simulink library "WBCLibrary"  (Simulink 7.9)
settings: Solver=ode45  StartTime=0.0  StopTime=10.0  RelTol=1e-3
undefined symbols (not defined in the file or in its folder): localName, robotName
libraries: WBCLibrary x5, dspmtrx3 x3, simulink x1, dspsigops x1
settings Model: ForwardingTableString=||__slOldName__||WBCLibrary/wholeBodyModel/Jacobians/COM Jacobian||__slNewName__||WBCLibrary/wholeBodyModel/Jacobians/Center of Mass Jacobian||__slOldName__||WBCLibrary/wholeBodyModel/Jacobians/Right Foot Jacobian1||__slNewName__||WBCLibrary/wholeBodyModel/Jacobians/Right Foot Jacobian||__slOldName__||WBCLibrary/wholeBodyActuators/setVelDes1||__slNewName__||WBCLibrary/wholeBodyActuators/Set Velocities||__slOldName__||WBCLibrary/wholeBodyActuators/setVelDes||__slNewName__||WBCLibrary/wholeBodyActuators/Set Velocities  Creator=jorhabib  LastModifiedBy=jorhabib

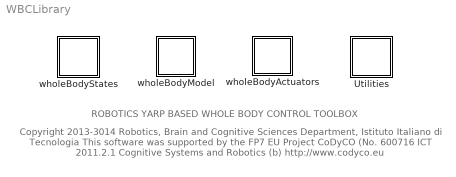
== system WBCLibrary ==
  note: ROBOTICS YARP BASED WHOLE BODY CONTROL TOOLBOX
  note: Copyright  2013-3014 Robotics, Brain and Cognitive Sciences Department, Istituto Italiano di Tecnologia
      | This software was supported by the FP7 EU Project CoDyCO (No. 600716 ICT 2011.2.1 Cognitive Systems and Robotics (b)
      | http://www.codyco.eu
  Utilities : Subsystem
      mask Display: image(imread('utilities.bmp'))
  wholeBodyActuators : Subsystem
      mask Display: image(imread('wholeBodyActuators.bmp'),'center')
  wholeBodyModel : Subsystem
      mask Display: image(imread('wholeBodyModel.bmp'),'center')
  wholeBodyStates : Subsystem
      mask Display: image(imread('wholeBodyStates.bmp'),'center');

== system WBCLibrary/Utilities ==
  DampPinv : Subsystem  mask{tol=1e-4}
      mask prompts: tol "Tolerance"
  S-Function : S-Function  FunctionName=sfun_time  Parameters=rate  EnableBusSupport=off  mask(Soft Real Time){rate=0.010}
      mask prompts: rate "Simulation rate"
      mask Display: disp('SoftRealTime')
  TruncPinv : Subsystem  mask{tol=1e-4}
      mask prompts: tol "Tolerance"
  WBI to yarp : Subsystem
  baseVelocity : Subsystem
      mask Type: baseVelocity
      mask Description: This block computes the velocity of the floating base of a bipedal robot
  errors : Subsystem
  holder : Subsystem
  minJerkTrajGen : Subsystem
      mask Type: minJerkTrajGen
      mask Description:
      | This block wraps the minJerkTrajGen class from iCub::ctrl::minJerkTrajGen.
      | 
      | The min jerk trajectory is approximated using a 3rd order LTI dynamical system (for more details see Pattacini2010). Position, velocity and acceleration trajectories are computed. The main advantage with respect to the standard polynomial form is that if the reference value yd changes there is no need to recompute the filter coefficients.
  yarp read : S-Function  FunctionName=yRead  Parameters=from,to,num  EnableBusSupport=off  mask{from=['/' robotName '/torso/state:o'], to='...', num=3}
  yarp to WBI : Subsystem
  yarp write : Subsystem  mask{port_name='...'}
      mask prompts: port_name "Specify port name starting with "/" e.g. '/port/input:i'"

== system WBCLibrary/wholeBodyActuators ==
  note: DO NOT USE YET.
      | UNDER DEVELOPMENT
  ControlMode : Subsystem  mask{ctrlMode=Velocity}
      mask prompts: ctrlMode "Control Mode"
      mask init:
      | switch ctrlMode
      |     case 'Velocity'
      | %         display('Velocity Mode selected')
      |         current = gcb;
      |         block = find_system(current,...
      |             'LookUnderMasks','on',...
      |             'FollowLinks','on','Name','set Velocities');
      |         if ~isempty(block)
      | %             display('setVelDes will be deleted')
      |             delete_block(block)
      | %             display('setVelDes has been deleted')
      |             add_block('WBCLibrary/wholeBodyActuators/set Velocities', [current,'/setVelDes1'])            
      | %             display('New setVelDes has been created')
      |             add_line(current,'In1/1',[current '/set Velocities/1'])
      |         else
      | %             display('A new setVelDes will be created')
      |             add_block('WBCLibrary/wholeBodyActuators/set Velocities', [current,'/setVelDes1'])            
      |         end
      | end
      mask StyleString: popup(Position|Velocity|Torque)
  Set Angles : Subsystem  mask{val=5, robotName=robotName, localName=localName}
      mask prompts: val "Block type"; robotName "Robot name"; localName "Local name"
  Set Torques : Subsystem  mask{val=6, robotName=robotName, localName=localName}
      mask prompts: val "Block type"; robotName "Robot name"; localName "Local name"
  Set Velocities : Subsystem  mask{val=4, robotName=robotName, localName=localName}
      mask prompts: val "Block type"; robotName "Robot name"; localName "Local name"

== system WBCLibrary/wholeBodyModel ==
  Dynamics : Subsystem
      mask Display: image(imread('dynamics.jpg'))
  Forward Kinematics : Subsystem
      mask Display: image(imread('rightLeg.jpg'))
  Jacobians : Subsystem
      mask Display: image(imread('jacobian.png'))
  Joint Limits : Subsystem  mask{robotName=robotName, localName=localName}
      mask prompts: robotName "Robot name"; localName "Local name"

== system WBCLibrary/wholeBodyStates ==
  DUMMY Joint Torques : Subsystem  mask{robotName=robotName, localName=localName}
      mask prompts: robotName "Robot name"; localName "Local name"
      mask Display: disp('dummy tau')
  Joint Accelerations : Subsystem  mask(Get Joint Accelerations){robotName=robotName, localName=localName}
      mask prompts: robotName "Robot name"; localName "Local name"
      mask Display: disp('ddq')
  Joint Angles : Subsystem  mask{robotName=robotName, localName=localName}
      mask Display: disp('q')
  Joint Torques : Subsystem  mask(Get Joint Torques){robotName=robotName, localName=localName}
      mask prompts: robotName "Robot name"; localName "Local name"
      mask Display: disp('tau')
  Joint Velocities : Subsystem  mask{robotName=robotName, localName=localName}
      mask Display: disp('dq')

== system WBCLibrary/Utilities/DampPinv ==
  mat : Inport
  sigma : Inport  Port=2
  Damped Pseudo Inverse : MATLAB Function  TreatAsAtomicUnit=on
  DPinv : Outport
  wires:
  sigma/1 -> Damped Pseudo Inverse/2(sigma)
  Damped Pseudo Inverse/1(DPinv) -> DPinv/1
  mat/1 -> Damped Pseudo Inverse/1(mat)

== system WBCLibrary/Utilities/TruncPinv ==
  S : Inport
  tol : Inport  Port=2
  Truncated PseudoInverse : MATLAB Function  TreatAsAtomicUnit=on
  Tpinv : Outport
  wires:
  S/1 -> Truncated PseudoInverse/1(mat)
  Truncated PseudoInverse/1(TPinv) -> Tpinv/1
  tol/1 -> Truncated PseudoInverse/2(tol)

== system WBCLibrary/Utilities/WBI to yarp ==
  WBI ordered : Inport
  Selector : Selector  InputPortWidth=25  IndexOptions=Index vector (dialog)  Indices=[1 2 3]  OutputSizes=1
  Selector1 : Selector  InputPortWidth=25  IndexOptions=Index vector (dialog)  Indices=[4 5 6 7 8]  OutputSizes=1
  Selector2 : Selector  InputPortWidth=25  IndexOptions=Index vector (dialog)  Indices=[9 10 11 12 13]  OutputSizes=1
  Selector3 : Selector  InputPortWidth=25  IndexOptions=Index vector (dialog)  Indices=[14 15 16 17 18 19]  OutputSizes=1
  Selector4 : Selector  InputPortWidth=25  IndexOptions=Index vector (dialog)  Indices=[20 21 22 23 24 25]  OutputSizes=1
  Selector5 : Selector  InputPortWidth=3  IndexOptions=Index vector (dialog)  Indices=[3 2 1]  OutputSizes=1
  torso : Outport
  leftArm : Outport  Port=2
  rightArm : Outport  Port=3
  leftLeg : Outport  Port=4
  rightLeg : Outport  Port=5
  wires:
  Selector1/1 -> leftArm/1
  Selector2/1 -> rightArm/1
  Selector3/1 -> leftLeg/1
  Selector4/1 -> rightLeg/1
  WBI ordered/1 -> Selector/1, Selector1/1, Selector2/1, Selector4/1, Selector3/1
  Selector/1 -> Selector5/1
  Selector5/1 -> torso/1

== system WBCLibrary/Utilities/baseVelocity ==
  JacobRF : Inport
  JacobLF : Inport  Port=2
  dq : Inport  Port=3
  MATLAB Function : MATLAB Function  TreatAsAtomicUnit=on
  baseVel : Outport
  wires:
  dq/1 -> MATLAB Function/3(qD)
  MATLAB Function/1(y) -> baseVel/1
  JacobRF/1 -> MATLAB Function/1(JacobRF)
  JacobLF/1 -> MATLAB Function/2(JacobLF)

== system WBCLibrary/Utilities/errors ==
  x : Inport
  y : Inport  Port=2
  Add : Sum  Inputs=+-
  Divide : Product  Inputs=*/
  x-y : Outport
  (x-y)./y : Outport  Port=2
  wires:
  Add/1 -> Divide/1, x-y/1
  x/1 -> Add/1
  y/1 -> Add/2, Divide/2
  Divide/1 -> (x-y)./y/1

== system WBCLibrary/Utilities/holder ==
  s : Inport
  Clock : Clock
  Compare To Constant : simulink/Logic and Bit Operations/Compare To Constant  relop===  const=0  OutDataTypeStr=boolean
  Memory : Memory
  Sample and Hold : dspsigops/Sample and Hold  trig=Falling edge  initCond=0  latchinput=off
  Switch : Switch  Criteria=u2 > Threshold
  s(0) : Outport
  wires:
  s/1 -> Switch/1, Memory/1
  Clock/1 -> Compare To Constant/1
  Compare To Constant/1 -> Sample and Hold/Trigger, Switch/2
  Sample and Hold/1 -> Switch/3
  Switch/1 -> s(0)/1
  Memory/1 -> Sample and Hold/1

== system WBCLibrary/Utilities/minJerkTrajGen ==
  desiredPos : Inport
  initPos : Inport  Port=2
  S-Function : S-Function  FunctionName=minJerkGenerator  Parameters=dim, rate, tt  EnableBusSupport=off  mask{dim=25, rate=10, tt=4}
      mask prompts: dim "Trajectory dimension (int)"; rate "Simulation rate (int) [ms]"; tt "Trajectory time [s]"
  pos : Outport
  vel : Outport  Port=2
  acc : Outport  Port=3
  wires:
  desiredPos/1 -> S-Function/2
  initPos/1 -> S-Function/1
  S-Function/3 -> acc/1
  S-Function/1 -> pos/1
  S-Function/2 -> vel/1

== system WBCLibrary/Utilities/yarp to WBI ==
  torso : Inport
  leftArm : Inport  Port=2
  rightArm : Inport  Port=3
  leftLeg : Inport  Port=4
  rightLeg : Inport  Port=5
  Mux3 : Mux  Inputs=5
  Selector : Selector  InputPortWidth=3  IndexOptions=Index vector (dialog)  Indices=[3 2 1]  OutputSizes=1
  WBI ordered : Outport
  wires:
  Selector/1 -> Mux3/1
  torso/1 -> Selector/1
  leftArm/1 -> Mux3/2
  rightArm/1 -> Mux3/3
  Mux3/1 -> WBI ordered/1
  leftLeg/1 -> Mux3/4
  rightLeg/1 -> Mux3/5

== system WBCLibrary/Utilities/yarp write ==
  In1 : Inport
  S-Function : S-Function  FunctionName=yWrite  Parameters=port_name  EnableBusSupport=off
  wires:
  In1/1 -> S-Function/1

== system WBCLibrary/wholeBodyActuators/ControlMode ==
  In1 : Inport

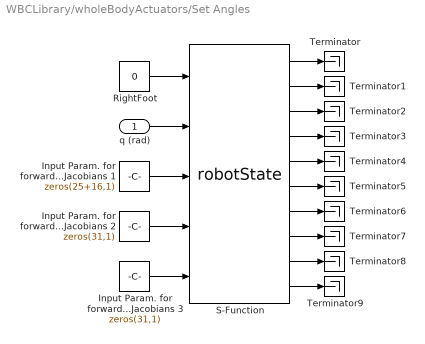
== system WBCLibrary/wholeBodyActuators/Set Angles ==
  q (rad) : Inport
  Input Param. for forwardKinematics and  computeJacobians 1 : Constant  Value=zeros(25+16,1)  OutDataTypeStr=double  SampleTime=-1
  Input Param. for forwardKinematics and  computeJacobians 2 : Constant  Value=zeros(31,1)  OutDataTypeStr=double  SampleTime=-1
  Input Param. for forwardKinematics and  computeJacobians 3 : Constant  Value=zeros(31,1)  OutDataTypeStr=double  SampleTime=-1
  RightFoot : Constant  Value=0  OutDataTypeStr=int8  SampleTime=-1
  S-Function : S-Function  FunctionName=robotState  Parameters=val,robotName,localName  EnableBusSupport=off
  Terminator{,1..9} (10 alike) : Terminator
  wires:
  RightFoot/1 -> S-Function/1
  q (rad)/1 -> S-Function/2
  S-Function/7 -> Terminator6/1
  S-Function/1 -> Terminator/1
  S-Function/2 -> Terminator1/1
  S-Function/3 -> Terminator2/1
  S-Function/4 -> Terminator3/1
  S-Function/5 -> Terminator4/1
  S-Function/6 -> Terminator5/1
  S-Function/8 -> Terminator7/1
  S-Function/9 -> Terminator8/1
  S-Function/10 -> Terminator9/1
  Input Param. for forwardKinematics and  computeJacobians 1/1 -> S-Function/3
  Input Param. for forwardKinematics and  computeJacobians 2/1 -> S-Function/4
  Input Param. for forwardKinematics and  computeJacobians 3/1 -> S-Function/5

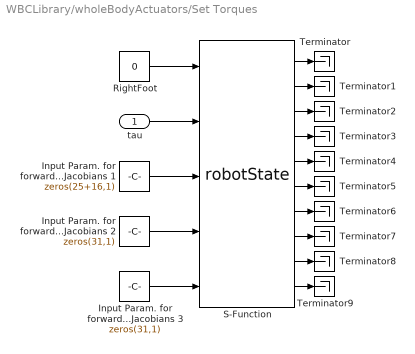
== system WBCLibrary/wholeBodyActuators/Set Torques ==
  tau : Inport
  Input Param. for forwardKinematics and  computeJacobians 1 : Constant  Value=zeros(25+16,1)  OutDataTypeStr=double  SampleTime=-1
  Input Param. for forwardKinematics and  computeJacobians 2 : Constant  Value=zeros(31,1)  OutDataTypeStr=double  SampleTime=-1
  Input Param. for forwardKinematics and  computeJacobians 3 : Constant  Value=zeros(31,1)  OutDataTypeStr=double  SampleTime=-1
  RightFoot : Constant  Value=0  OutDataTypeStr=int8  SampleTime=-1
  S-Function : S-Function  FunctionName=robotState  Parameters=val,robotName,localName  EnableBusSupport=off
  Terminator{,1..9} (10 alike) : Terminator
  wires:
  S-Function/6 -> Terminator5/1
  S-Function/5 -> Terminator4/1
  S-Function/4 -> Terminator3/1
  S-Function/3 -> Terminator2/1
  S-Function/2 -> Terminator1/1
  S-Function/1 -> Terminator/1
  S-Function/7 -> Terminator6/1
  tau/1 -> S-Function/2
  RightFoot/1 -> S-Function/1
  S-Function/9 -> Terminator8/1
  S-Function/8 -> Terminator7/1
  S-Function/10 -> Terminator9/1
  Input Param. for forwardKinematics and  computeJacobians 1/1 -> S-Function/3
  Input Param. for forwardKinematics and  computeJacobians 2/1 -> S-Function/4
  Input Param. for forwardKinematics and  computeJacobians 3/1 -> S-Function/5

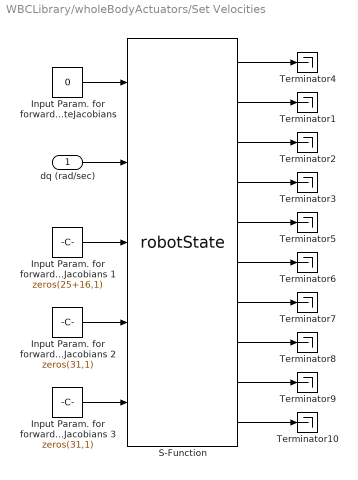
== system WBCLibrary/wholeBodyActuators/Set Velocities ==
  dq (rad/sec) : Inport
  "Input Param. for forwardKinematics and  computeJacobians " : Constant  Value=0  OutDataTypeStr=int8
  Input Param. for forwardKinematics and  computeJacobians 1 : Constant  Value=zeros(25+16,1)  OutDataTypeStr=double  SampleTime=-1
  Input Param. for forwardKinematics and  computeJacobians 2 : Constant  Value=zeros(31,1)  OutDataTypeStr=double  SampleTime=-1
  Input Param. for forwardKinematics and  computeJacobians 3 : Constant  Value=zeros(31,1)  OutDataTypeStr=double  SampleTime=-1
  S-Function : S-Function  FunctionName=robotState  Parameters=val,robotname,localname  EnableBusSupport=off  mask{val=val, robotname=robotName, localname=localName}
      mask prompts: val "Value"; robotname "Robot Name (icub - icubSim)"; localname "Module Name"
  Terminator{1..10} (10 alike) : Terminator
  wires:
  S-Function/4 -> Terminator3/1
  "Input Param. for forwardKinematics and  computeJacobians "/1 -> S-Function/1
  S-Function/3 -> Terminator2/1
  S-Function/1 -> Terminator4/1
  S-Function/2 -> Terminator1/1
  dq (rad/sec)/1 -> S-Function/2
  S-Function/5 -> Terminator5/1
  S-Function/6 -> Terminator6/1
  S-Function/7 -> Terminator7/1
  S-Function/8 -> Terminator8/1
  S-Function/9 -> Terminator9/1
  S-Function/10 -> Terminator10/1
  Input Param. for forwardKinematics and  computeJacobians 1/1 -> S-Function/3
  Input Param. for forwardKinematics and  computeJacobians 2/1 -> S-Function/4
  Input Param. for forwardKinematics and  computeJacobians 3/1 -> S-Function/5

== system WBCLibrary/wholeBodyModel/Dynamics ==
  Cent Momentum : Subsystem
  Inverse Dynamics : Subsystem  mask(Inverse Dynamics){robotName=robotName, localName=localName}
      mask prompts: robotName "Robot name"; localName "Local name"
  computeh : Subsystem  mask{val=7, robotname=robotName, localname=localName}
      mask prompts: val "Block type"; robotname "Robot name"; localname "Module name"
  dJ*dq LeftFoot : Subsystem  mask{val=9, robotName=robotName, localName=localName}
      mask prompts: val "Block type"; robotName "Robot name"; localName "Local name"
      mask init:
      | val = 9
      | robotName = 'icubSim'
      | localName = 'simulink'
  dJ*dq RightFoot : Subsystem  mask{val=9, robotName=robotName, localName=localName}
      mask prompts: val "Block type"; robotName "Robot name"; localName "Local name"
      mask init:
      | val = 9
      | robotName = 'icubSim'
      | localName = 'simulink'
  massMatrix : Subsystem  mask{val=8, robotname=robotName, localname=localName}
      mask prompts: val "Block type"; robotname "Robot name"; localname "Module name"

== system WBCLibrary/wholeBodyModel/Forward Kinematics ==
  "COMFwdKin " : Subsystem  mask{robotName=robotName, localName=localName}
      mask prompts: robotName "robot name"; localName "local name"
  LeftFootFwdKin : Subsystem  mask{robotName=robotName, localName=localName}
      mask prompts: robotName "robot name"; localName "local name"
  RightFootFwdKin : Subsystem  mask{robotName=robotName, localName=localName}
      mask prompts: robotName "robot name"; localName "local name"

== system WBCLibrary/wholeBodyModel/Jacobians ==
  Center of Mass Jacobian : Subsystem  mask{robotName=robotName, localName=localName}
      mask prompts: robotName "robot name"; localName "local name"
  Left Foot Jacobian : Subsystem  mask{robotName=robotName, localName=localName}
      mask prompts: robotName "robot name"; localName "local name"
  Right Foot Jacobian : Subsystem  mask{robotName=robotName, localName=localName}
      mask prompts: robotName "robot name"; localName "local name"

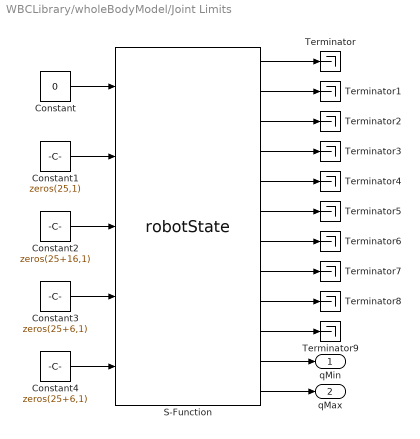
== system WBCLibrary/wholeBodyModel/Joint Limits ==
  Constant : Constant  Value=0  OutDataTypeStr=int8  SampleTime=-1
  Constant1 : Constant  Value=zeros(25,1)  OutDataTypeStr=double  SampleTime=-1
  Constant2 : Constant  Value=zeros(25+16,1)  OutDataTypeStr=double  SampleTime=-1
  Constant3 : Constant  Value=zeros(25+6,1)  OutDataTypeStr=double  SampleTime=-1
  Constant4 : Constant  Value=zeros(25+6,1)  OutDataTypeStr=double  SampleTime=-1
  S-Function : S-Function  FunctionName=robotState  Parameters=13,robotName,localName  EnableBusSupport=off
  Terminator{,1..9} (10 alike) : Terminator
  qMin : Outport
  qMax : Outport  Port=2
  wires:
  S-Function/12 -> qMax/1
  S-Function/11 -> qMin/1
  S-Function/10 -> Terminator9/1
  S-Function/9 -> Terminator8/1
  S-Function/8 -> Terminator7/1
  S-Function/7 -> Terminator6/1
  S-Function/6 -> Terminator5/1
  S-Function/5 -> Terminator4/1
  S-Function/4 -> Terminator3/1
  S-Function/3 -> Terminator2/1
  S-Function/2 -> Terminator1/1
  S-Function/1 -> Terminator/1
  Constant4/1 -> S-Function/5
  Constant3/1 -> S-Function/4
  Constant2/1 -> S-Function/3
  Constant1/1 -> S-Function/2
  Constant/1 -> S-Function/1

== system WBCLibrary/wholeBodyStates/DUMMY Joint Torques ==
  tau from ports : Subsystem
  yarp to WBI : Subsystem
  joint tau : Outport
  wires:
  tau from ports/2(leftArm) -> yarp to WBI/2(leftArm)
  tau from ports/1(torso) -> yarp to WBI/1(torso)
  tau from ports/5(rightLeg) -> yarp to WBI/5(rightLeg)
  tau from ports/3(rightArm) -> yarp to WBI/3(rightArm)
  tau from ports/4(leftLeg) -> yarp to WBI/4(leftLeg)
  yarp to WBI/1(WBI ordered) -> joint tau/1

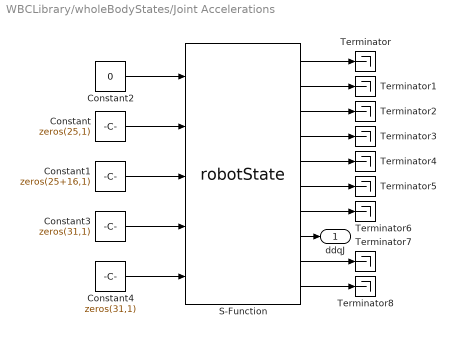
== system WBCLibrary/wholeBodyStates/Joint Accelerations ==
  Constant : Constant  Value=zeros(25,1)  OutDataTypeStr=double  SampleTime=-1
  Constant1 : Constant  Value=zeros(25+16,1)  OutDataTypeStr=double  SampleTime=-1
  Constant2 : Constant  Value=0  OutDataTypeStr=int8  SampleTime=-1
  Constant3 : Constant  Value=zeros(31,1)  OutDataTypeStr=double  SampleTime=-1
  Constant4 : Constant  Value=zeros(31,1)  OutDataTypeStr=double  SampleTime=-1
  S-Function : S-Function  FunctionName=robotState  Parameters=10,robotName,localName  EnableBusSupport=off
  Terminator{,1..8} (9 alike) : Terminator
  ddqJ : Outport
  wires:
  S-Function/8 -> ddqJ/1
  S-Function/10 -> Terminator8/1
  S-Function/9 -> Terminator7/1
  S-Function/7 -> Terminator6/1
  S-Function/6 -> Terminator5/1
  S-Function/5 -> Terminator4/1
  S-Function/4 -> Terminator3/1
  S-Function/3 -> Terminator2/1
  S-Function/2 -> Terminator1/1
  S-Function/1 -> Terminator/1
  Constant4/1 -> S-Function/5
  Constant3/1 -> S-Function/4
  Constant1/1 -> S-Function/3
  Constant2/1 -> S-Function/1
  Constant/1 -> S-Function/2

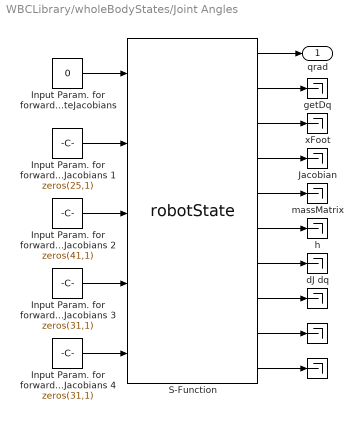
== system WBCLibrary/wholeBodyStates/Joint Angles ==
  " " : Terminator
  "  " : Terminator
  "   " : Terminator
  "Input Param. for forwardKinematics and  computeJacobians " : Constant  Value=0  OutDataTypeStr=int8
  Input Param. for forwardKinematics and  computeJacobians 1 : Constant  Value=zeros(25,1)  OutDataTypeStr=double  SampleTime=-1
  Input Param. for forwardKinematics and  computeJacobians 2 : Constant  Value=zeros(41,1)  OutDataTypeStr=double  SampleTime=-1
  Input Param. for forwardKinematics and  computeJacobians 3 : Constant  Value=zeros(31,1)  OutDataTypeStr=double  SampleTime=-1
  Input Param. for forwardKinematics and  computeJacobians 4 : Constant  Value=zeros(31,1)  OutDataTypeStr=double  SampleTime=-1
  Jacobian : Terminator
  S-Function : S-Function  FunctionName=robotState  Parameters=val,robotname,localname  EnableBusSupport=off  mask{val=0, robotname=robotName, localname=localName}
      mask prompts: val "Value"; robotname "Robot Name (icub - icubSim)"; localname "Module Name"
  dJ dq : Terminator
  getDq : Terminator
  h : Terminator
  massMatrix : Terminator
  xFoot : Terminator
  qrad : Outport
  wires:
  Input Param. for forwardKinematics and  computeJacobians 1/1 -> S-Function/2
  S-Function/2 -> getDq/1
  S-Function/1 -> qrad/1
  S-Function/3 -> xFoot/1
  "Input Param. for forwardKinematics and  computeJacobians "/1 -> S-Function/1
  S-Function/4 -> Jacobian/1
  S-Function/5 -> massMatrix/1
  S-Function/6 -> h/1
  S-Function/7 -> dJ dq/1
  S-Function/8 -> " "/1
  S-Function/9 -> "  "/1
  S-Function/10 -> "   "/1
  Input Param. for forwardKinematics and  computeJacobians 2/1 -> S-Function/3
  Input Param. for forwardKinematics and  computeJacobians 3/1 -> S-Function/4
  Input Param. for forwardKinematics and  computeJacobians 4/1 -> S-Function/5

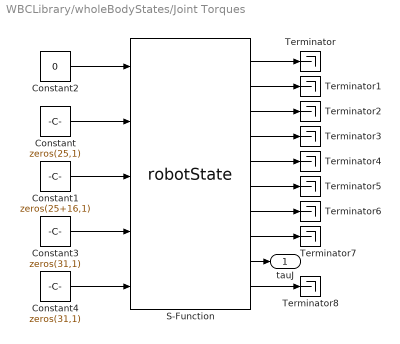
== system WBCLibrary/wholeBodyStates/Joint Torques ==
  Constant : Constant  Value=zeros(25,1)  OutDataTypeStr=double  SampleTime=-1
  Constant1 : Constant  Value=zeros(25+16,1)  OutDataTypeStr=double  SampleTime=-1
  Constant2 : Constant  Value=0  OutDataTypeStr=int8  SampleTime=-1
  Constant3 : Constant  Value=zeros(31,1)  OutDataTypeStr=double  SampleTime=-1
  Constant4 : Constant  Value=zeros(31,1)  OutDataTypeStr=double  SampleTime=-1
  S-Function : S-Function  FunctionName=robotState  Parameters=11,robotName,localName  EnableBusSupport=off
  Terminator{,1..8} (9 alike) : Terminator
  tauJ : Outport
  wires:
  S-Function/10 -> Terminator8/1
  S-Function/8 -> Terminator7/1
  S-Function/7 -> Terminator6/1
  S-Function/6 -> Terminator5/1
  S-Function/5 -> Terminator4/1
  S-Function/4 -> Terminator3/1
  S-Function/3 -> Terminator2/1
  S-Function/2 -> Terminator1/1
  S-Function/1 -> Terminator/1
  S-Function/9 -> tauJ/1
  Constant4/1 -> S-Function/5
  Constant3/1 -> S-Function/4
  Constant1/1 -> S-Function/3
  Constant2/1 -> S-Function/1
  Constant/1 -> S-Function/2

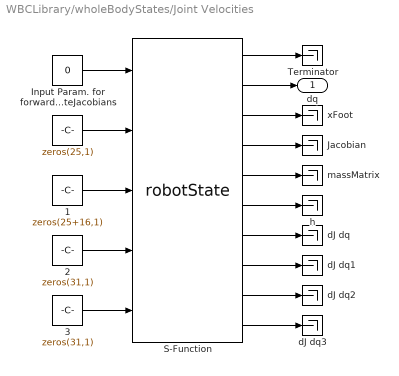
== system WBCLibrary/wholeBodyStates/Joint Velocities ==
  " " : Constant  Value=zeros(25,1)  OutDataTypeStr=double  SampleTime=-1
  " 1" : Constant  Value=zeros(25+16,1)  OutDataTypeStr=double  SampleTime=-1
  " 2" : Constant  Value=zeros(31,1)  OutDataTypeStr=double  SampleTime=-1
  " 3" : Constant  Value=zeros(31,1)  OutDataTypeStr=double  SampleTime=-1
  "Input Param. for forwardKinematics and  computeJacobians " : Constant  Value=0  OutDataTypeStr=int8
  Jacobian : Terminator
  S-Function : S-Function  FunctionName=robotState  Parameters=val,robotname,localname  EnableBusSupport=off  mask{val=1, robotname=robotName, localname=localName}
      mask prompts: val "Value"; robotname "Robot Name (icub - icubSim)"; localname "Module Name"
  Terminator : Terminator
  dJ dq{,1..3} (4 alike) : Terminator
  h : Terminator
  massMatrix : Terminator
  xFoot : Terminator
  dq : Outport
  wires:
  " "/1 -> S-Function/2
  S-Function/2 -> dq/1
  S-Function/1 -> Terminator/1
  S-Function/3 -> xFoot/1
  "Input Param. for forwardKinematics and  computeJacobians "/1 -> S-Function/1
  S-Function/4 -> Jacobian/1
  S-Function/5 -> massMatrix/1
  S-Function/6 -> h/1
  S-Function/7 -> dJ dq/1
  S-Function/8 -> dJ dq1/1
  S-Function/9 -> dJ dq2/1
  S-Function/10 -> dJ dq3/1
  " 1"/1 -> S-Function/3
  " 2"/1 -> S-Function/4
  " 3"/1 -> S-Function/5

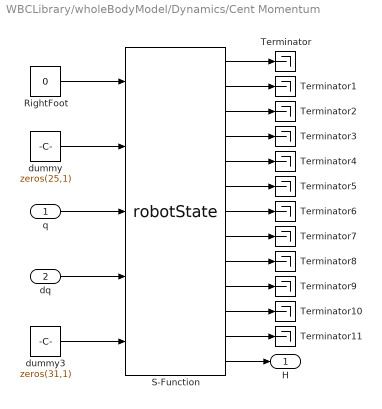
== system WBCLibrary/wholeBodyModel/Dynamics/Cent Momentum ==
  q : Inport
  dq : Inport  Port=2
  RightFoot : Constant  Value=0  OutDataTypeStr=int8  SampleTime=-1
  S-Function : S-Function  FunctionName=robotState  Parameters=14,robotName,localName  EnableBusSupport=off
  Terminator{,1..11} (12 alike) : Terminator
  dummy : Constant  Value=zeros(25,1)  OutDataTypeStr=double  SampleTime=-1
  dummy3 : Constant  Value=zeros(31,1)  OutDataTypeStr=double  SampleTime=-1
  H : Outport
  wires:
  S-Function/13 -> H/1
  dummy3/1 -> S-Function/5
  dq/1 -> S-Function/4
  q/1 -> S-Function/3
  dummy/1 -> S-Function/2
  RightFoot/1 -> S-Function/1
  S-Function/12 -> Terminator11/1
  S-Function/11 -> Terminator10/1
  S-Function/10 -> Terminator9/1
  S-Function/9 -> Terminator8/1
  S-Function/8 -> Terminator7/1
  S-Function/7 -> Terminator6/1
  S-Function/6 -> Terminator5/1
  S-Function/5 -> Terminator4/1
  S-Function/4 -> Terminator3/1
  S-Function/3 -> Terminator2/1
  S-Function/2 -> Terminator1/1
  S-Function/1 -> Terminator/1

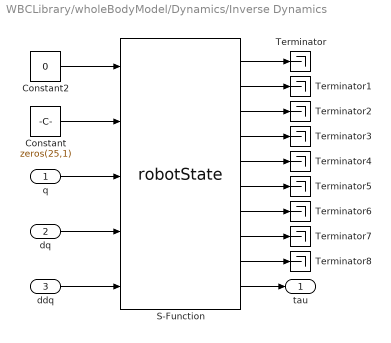
== system WBCLibrary/wholeBodyModel/Dynamics/Inverse Dynamics ==
  q : Inport
  dq : Inport  Port=2
  ddq : Inport  Port=3
  Constant : Constant  Value=zeros(25,1)  OutDataTypeStr=double  SampleTime=-1
  Constant2 : Constant  Value=0  OutDataTypeStr=int8  SampleTime=-1
  S-Function : S-Function  FunctionName=robotState  Parameters=12,robotName,localName  EnableBusSupport=off
  Terminator{,1..8} (9 alike) : Terminator
  tau : Outport
  wires:
  S-Function/10 -> tau/1
  S-Function/9 -> Terminator8/1
  Constant/1 -> S-Function/2
  Constant2/1 -> S-Function/1
  q/1 -> S-Function/3
  dq/1 -> S-Function/4
  ddq/1 -> S-Function/5
  S-Function/1 -> Terminator/1
  S-Function/2 -> Terminator1/1
  S-Function/3 -> Terminator2/1
  S-Function/4 -> Terminator3/1
  S-Function/5 -> Terminator4/1
  S-Function/6 -> Terminator5/1
  S-Function/7 -> Terminator6/1
  S-Function/8 -> Terminator7/1

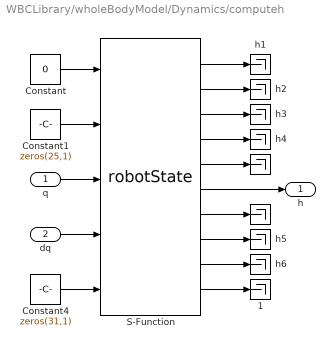
== system WBCLibrary/wholeBodyModel/Dynamics/computeh ==
  q : Inport
  dq : Inport  Port=2
  " " : Terminator
  "  " : Terminator
  "  1" : Terminator
  Constant : Constant  Value=0  OutDataTypeStr=int8  SampleTime=-1
  Constant1 : Constant  Value=zeros(25,1)  OutDataTypeStr=double  SampleTime=-1
  Constant4 : Constant  Value=zeros(31,1)  OutDataTypeStr=double  SampleTime=-1
  S-Function : S-Function  FunctionName=robotState  Parameters=val,robotname,localname  EnableBusSupport=off
  h{1..6} (6 alike) : Terminator
  h : Outport
  wires:
  Constant/1 -> S-Function/1
  Constant1/1 -> S-Function/2
  S-Function/1 -> h1/1
  S-Function/2 -> h2/1
  S-Function/3 -> h3/1
  S-Function/4 -> h4/1
  S-Function/5 -> "  "/1
  S-Function/7 -> " "/1
  S-Function/6 -> h/1
  S-Function/8 -> h5/1
  S-Function/9 -> h6/1
  S-Function/10 -> "  1"/1
  q/1 -> S-Function/3
  dq/1 -> S-Function/4
  Constant4/1 -> S-Function/5

== system WBCLibrary/wholeBodyModel/Dynamics/dJ*dq LeftFoot ==
  q : Inport
  dq : Inport  Port=2
  LeftFoot : Constant  OutDataTypeStr=int8  SampleTime=-1
  S-Function : S-Function  FunctionName=robotState  Parameters=val,robotName,localName  EnableBusSupport=off
  Terminator{,1..8} (9 alike) : Terminator
  dummy : Constant  Value=zeros(25,1)  OutDataTypeStr=double  SampleTime=-1
  dummy3 : Constant  Value=zeros(31,1)  OutDataTypeStr=double  SampleTime=-1
  dJdq : Outport
  wires:
  S-Function/6 -> Terminator5/1
  S-Function/5 -> Terminator4/1
  S-Function/4 -> Terminator3/1
  S-Function/3 -> Terminator2/1
  S-Function/2 -> Terminator1/1
  S-Function/1 -> Terminator/1
  S-Function/7 -> dJdq/1
  dummy/1 -> S-Function/2
  LeftFoot/1 -> S-Function/1
  S-Function/8 -> Terminator6/1
  S-Function/9 -> Terminator7/1
  S-Function/10 -> Terminator8/1
  q/1 -> S-Function/3
  dq/1 -> S-Function/4
  dummy3/1 -> S-Function/5

== system WBCLibrary/wholeBodyModel/Dynamics/dJ*dq RightFoot ==
  q : Inport
  dq : Inport  Port=2
  RightFoot : Constant  Value=0  OutDataTypeStr=int8  SampleTime=-1
  S-Function : S-Function  FunctionName=robotState  Parameters=val,robotName,localName  EnableBusSupport=off
  Terminator{,1..8} (9 alike) : Terminator
  dummy : Constant  Value=zeros(25,1)  OutDataTypeStr=double  SampleTime=-1
  dummy3 : Constant  Value=zeros(31,1)  OutDataTypeStr=double  SampleTime=-1
  dJdq : Outport
  wires:
  S-Function/6 -> Terminator5/1
  S-Function/5 -> Terminator4/1
  S-Function/4 -> Terminator3/1
  S-Function/3 -> Terminator2/1
  S-Function/2 -> Terminator1/1
  S-Function/1 -> Terminator/1
  S-Function/7 -> dJdq/1
  dummy/1 -> S-Function/2
  RightFoot/1 -> S-Function/1
  S-Function/8 -> Terminator6/1
  S-Function/9 -> Terminator7/1
  S-Function/10 -> Terminator8/1
  q/1 -> S-Function/3
  dq/1 -> S-Function/4
  dummy3/1 -> S-Function/5

== system WBCLibrary/wholeBodyModel/Dynamics/massMatrix ==
  q : Inport
  Reshape : Reshape  OutputDimensionality=Customize  OutputDimensions=[25+6,25+6]
  massMatrix : Subsystem
  M : Outport
  wires:
  Reshape/1 -> M/1
  massMatrix/1(massMatrix) -> Reshape/1
  q/1 -> massMatrix/1(q)

== system WBCLibrary/wholeBodyModel/Forward Kinematics/COMFwdKin  ==
  "Input Param. for forwardKinematics and  computeJacobians " : Constant  Value=2  OutDataTypeStr=int8  SampleTime=-1
  Input Param. for forwardKinematics and  computeJacobians 1 : Constant  Value=zeros(25,1)  OutDataTypeStr=double  SampleTime=-1
  Input Param. for forwardKinematics and  computeJacobians 2 : Constant  Value=zeros(25+16,1)  OutDataTypeStr=double  SampleTime=-1
  Input Param. for forwardKinematics and  computeJacobians 3 : Constant  Value=zeros(31,1)  OutDataTypeStr=double  SampleTime=-1
  Input Param. for forwardKinematics and  computeJacobians 4 : Constant  Value=zeros(31,1)  OutDataTypeStr=double  SampleTime=-1
  Jacobian : Terminator
  S-Function : S-Function  FunctionName=robotState  Parameters=val,robotname,localname  EnableBusSupport=off  mask{val=2, robotname=robotName, localname=localName}
      mask prompts: val "Value"; robotname "Robot Name (icub - icubSim)"; localname "Module Name"
  dJ dq{,1..3} (4 alike) : Terminator
  getDq : Terminator
  h : Terminator
  massMatrix : Terminator
  qrad : Terminator
  xCOM : Outport
  wires:
  S-Function/4 -> Jacobian/1
  "Input Param. for forwardKinematics and  computeJacobians "/1 -> S-Function/1
  S-Function/3 -> xCOM/1
  S-Function/1 -> qrad/1
  S-Function/2 -> getDq/1
  Input Param. for forwardKinematics and  computeJacobians 1/1 -> S-Function/2
  S-Function/5 -> massMatrix/1
  S-Function/6 -> h/1
  S-Function/7 -> dJ dq/1
  S-Function/8 -> dJ dq1/1
  S-Function/9 -> dJ dq2/1
  S-Function/10 -> dJ dq3/1
  Input Param. for forwardKinematics and  computeJacobians 2/1 -> S-Function/3
  Input Param. for forwardKinematics and  computeJacobians 3/1 -> S-Function/4
  Input Param. for forwardKinematics and  computeJacobians 4/1 -> S-Function/5

== system WBCLibrary/wholeBodyModel/Forward Kinematics/LeftFootFwdKin ==
  "Input Param. for forwardKinematics and  computeJacobians " : Constant  OutDataTypeStr=int8  SampleTime=-1
  Input Param. for forwardKinematics and  computeJacobians 1 : Constant  Value=zeros(25,1)  OutDataTypeStr=double  SampleTime=-1
  Input Param. for forwardKinematics and  computeJacobians 2 : Constant  Value=zeros(25+16,1)  OutDataTypeStr=double  SampleTime=-1
  Input Param. for forwardKinematics and  computeJacobians 3 : Constant  Value=zeros(31,1)  OutDataTypeStr=double  SampleTime=-1
  Input Param. for forwardKinematics and  computeJacobians 4 : Constant  Value=zeros(31,1)  OutDataTypeStr=double  SampleTime=-1
  Jacobian : Terminator
  S-Function : S-Function  FunctionName=robotState  Parameters=val,robotname,localname  EnableBusSupport=off  mask{val=2, robotname=robotName, localname=localName}
      mask prompts: val "Value"; robotname "Robot Name (icub - icubSim)"; localname "Module Name"
  dJ dq : Terminator
  getDq : Terminator
  h : Terminator
  massMatrix : Terminator
  qrad : Terminator
  xLeftFoot : Outport
  wires:
  S-Function/4 -> Jacobian/1
  "Input Param. for forwardKinematics and  computeJacobians "/1 -> S-Function/1
  S-Function/3 -> xLeftFoot/1
  S-Function/1 -> qrad/1
  S-Function/2 -> getDq/1
  Input Param. for forwardKinematics and  computeJacobians 1/1 -> S-Function/2
  S-Function/5 -> massMatrix/1
  S-Function/6 -> h/1
  S-Function/7 -> dJ dq/1
  Input Param. for forwardKinematics and  computeJacobians 2/1 -> S-Function/3
  Input Param. for forwardKinematics and  computeJacobians 3/1 -> S-Function/4
  Input Param. for forwardKinematics and  computeJacobians 4/1 -> S-Function/5

== system WBCLibrary/wholeBodyModel/Forward Kinematics/RightFootFwdKin ==
  "Input Param. for forwardKinematics and  computeJacobians " : Constant  Value=0  OutDataTypeStr=int8  SampleTime=-1
  Input Param. for forwardKinematics and  computeJacobians 1 : Constant  Value=zeros(25,1)  OutDataTypeStr=double  SampleTime=-1
  Input Param. for forwardKinematics and  computeJacobians 2 : Constant  Value=zeros(25+16,1)  OutDataTypeStr=double  SampleTime=-1
  Input Param. for forwardKinematics and  computeJacobians 3 : Constant  Value=zeros(31,1)  OutDataTypeStr=double  SampleTime=-1
  Input Param. for forwardKinematics and  computeJacobians 4 : Constant  Value=zeros(31,1)  OutDataTypeStr=double  SampleTime=-1
  Jacobian : Terminator
  S-Function : S-Function  FunctionName=robotState  Parameters=val,robotname,localname  EnableBusSupport=off  mask{val=2, robotname=robotName, localname=localName}
      mask prompts: val "Value"; robotname "Robot Name (icub - icubSim)"; localname "Module Name"
  dJ dq{,1..3} (4 alike) : Terminator
  getDq : Terminator
  h : Terminator
  massMatrix : Terminator
  qrad : Terminator
  xRightFoot : Outport
  wires:
  S-Function/7 -> dJ dq/1
  S-Function/6 -> h/1
  S-Function/5 -> massMatrix/1
  Input Param. for forwardKinematics and  computeJacobians 1/1 -> S-Function/2
  S-Function/2 -> getDq/1
  S-Function/1 -> qrad/1
  S-Function/3 -> xRightFoot/1
  "Input Param. for forwardKinematics and  computeJacobians "/1 -> S-Function/1
  S-Function/4 -> Jacobian/1
  S-Function/8 -> dJ dq1/1
  S-Function/9 -> dJ dq2/1
  S-Function/10 -> dJ dq3/1
  Input Param. for forwardKinematics and  computeJacobians 2/1 -> S-Function/3
  Input Param. for forwardKinematics and  computeJacobians 3/1 -> S-Function/4
  Input Param. for forwardKinematics and  computeJacobians 4/1 -> S-Function/5

== system WBCLibrary/wholeBodyModel/Jacobians/Center of Mass Jacobian ==
  Right Foot  Jacobian1 : Subsystem
  Transpose2 : dspmtrx3/Transpose  Hermitian=off  overflowFlag=off
  rs1 : Reshape  OutputDimensionality=Customize  OutputDimensions=[31,6]
  COMJacob : Outport
  wires:
  Transpose2/1 -> COMJacob/1
  rs1/1 -> Transpose2/1
  Right Foot  Jacobian1/1(Jacobian) -> rs1/1

== system WBCLibrary/wholeBodyModel/Jacobians/Left Foot Jacobian ==
  Left Foot  Jacobian1 : Subsystem
  Transpose1 : dspmtrx3/Transpose  Hermitian=off  overflowFlag=off
  rs2 : Reshape  OutputDimensionality=Customize  OutputDimensions=[31,6]
  LFootJacob : Outport
  wires:
  Left Foot  Jacobian1/1(Jacobian) -> rs2/1
  rs2/1 -> Transpose1/1
  Transpose1/1 -> LFootJacob/1

== system WBCLibrary/wholeBodyModel/Jacobians/Right Foot Jacobian ==
  Right Foot  Jacobian1 : Subsystem
  Transpose2 : dspmtrx3/Transpose  Hermitian=off  overflowFlag=off
  rs1 : Reshape  OutputDimensionality=Customize  OutputDimensions=[31,6]
  RFootJacob : Outport
  wires:
  Right Foot  Jacobian1/1(Jacobian) -> rs1/1
  rs1/1 -> Transpose2/1
  Transpose2/1 -> RFootJacob/1

== system WBCLibrary/wholeBodyStates/DUMMY Joint Torques/tau from ports ==
  Mux : Mux  Inputs=5
  Mux1 : Mux  Inputs=5
  Mux2 : Mux  Inputs=3
  Mux4 : Mux  Inputs=6
  Mux5 : Mux  Inputs=6
  yarp armL : WBCLibrary/Utilities/yarp read  from=['/' robotName '/left_arm/analog:o/torques']  to='...'  num=5
  yarp armR : WBCLibrary/Utilities/yarp read  from=['/' robotName '/right_arm/analog:o/torques']  to='...'  num=5
  yarp legL : WBCLibrary/Utilities/yarp read  from=['/' robotName '/left_leg/analog:o/torques']  to='...'  num=6
  yarp legR : WBCLibrary/Utilities/yarp read  from=['/' robotName '/right_leg/analog:o/torques']  to='...'  num=6
  yarp torso : WBCLibrary/Utilities/yarp read  from=['/' robotName '/torso/analog:o/torques']  to='...'  num=3
  torso : Outport
  leftArm : Outport  Port=2
  rightArm : Outport  Port=3
  leftLeg : Outport  Port=4
  rightLeg : Outport  Port=5
  wires:
  yarp legR/6 -> Mux4/6
  yarp legR/5 -> Mux4/5
  yarp legR/4 -> Mux4/4
  yarp legR/3 -> Mux4/3
  yarp legR/2 -> Mux4/2
  yarp legR/1 -> Mux4/1
  yarp legL/6 -> Mux5/6
  yarp legL/5 -> Mux5/5
  yarp legL/4 -> Mux5/4
  yarp legL/3 -> Mux5/3
  yarp legL/2 -> Mux5/2
  yarp legL/1 -> Mux5/1
  yarp armR/5 -> Mux/5
  yarp armR/4 -> Mux/4
  yarp armR/3 -> Mux/3
  yarp armR/2 -> Mux/2
  yarp armR/1 -> Mux/1
  yarp armL/5 -> Mux1/5
  yarp armL/4 -> Mux1/4
  yarp armL/3 -> Mux1/3
  yarp armL/2 -> Mux1/2
  yarp armL/1 -> Mux1/1
  yarp torso/1 -> Mux2/1
  yarp torso/2 -> Mux2/2
  yarp torso/3 -> Mux2/3
  Mux2/1 -> torso/1
  Mux1/1 -> leftArm/1
  Mux/1 -> rightArm/1
  Mux5/1 -> leftLeg/1
  Mux4/1 -> rightLeg/1

== system WBCLibrary/wholeBodyStates/DUMMY Joint Torques/yarp to WBI ==
  torso : Inport
  leftArm : Inport  Port=2
  rightArm : Inport  Port=3
  leftLeg : Inport  Port=4
  rightLeg : Inport  Port=5
  Mux3 : Mux  Inputs=5
  Selector : Selector  InputPortWidth=3  IndexOptions=Index vector (dialog)  Indices=[3 2 1]  OutputSizes=1
  WBI ordered : Outport
  wires:
  Selector/1 -> Mux3/1
  torso/1 -> Selector/1
  leftArm/1 -> Mux3/2
  rightArm/1 -> Mux3/3
  Mux3/1 -> WBI ordered/1
  leftLeg/1 -> Mux3/4
  rightLeg/1 -> Mux3/5

== system WBCLibrary/wholeBodyModel/Dynamics/massMatrix/massMatrix ==
  q : Inport
  Constant : Constant  Value=0  OutDataTypeStr=int8  SampleTime=-1
  Constant1 : Constant  Value=zeros(25,1)  OutDataTypeStr=double  SampleTime=-1
  Constant3 : Constant  Value=zeros(31,1)  OutDataTypeStr=double  SampleTime=-1
  Constant4 : Constant  Value=zeros(31,1)  OutDataTypeStr=double  SampleTime=-1
  S-Function : S-Function  FunctionName=robotState  Parameters=val,robotname,localname  EnableBusSupport=off
  Terminator{,1..8} (9 alike) : Terminator
  massMatrix : Outport
  wires:
  S-Function/7 -> Terminator5/1
  S-Function/6 -> Terminator4/1
  S-Function/4 -> Terminator3/1
  S-Function/3 -> Terminator2/1
  S-Function/2 -> Terminator1/1
  S-Function/1 -> Terminator/1
  S-Function/5 -> massMatrix/1
  Constant1/1 -> S-Function/2
  Constant/1 -> S-Function/1
  S-Function/8 -> Terminator6/1
  S-Function/9 -> Terminator7/1
  S-Function/10 -> Terminator8/1
  q/1 -> S-Function/3
  Constant3/1 -> S-Function/4
  Constant4/1 -> S-Function/5

== system WBCLibrary/wholeBodyModel/Jacobians/Center of Mass Jacobian/Right Foot  Jacobian1 ==
  "Input Param. for forwardKinematics and  computeJacobians " : Constant  Value=2  OutDataTypeStr=int8  SampleTime=-1
  Input Param. for forwardKinematics and  computeJacobians 1 : Constant  Value=zeros(25,1)  OutDataTypeStr=double  SampleTime=-1
  Input Param. for forwardKinematics and  computeJacobians 2 : Constant  Value=zeros(25+16,1)  OutDataTypeStr=double  SampleTime=-1
  Input Param. for forwardKinematics and  computeJacobians 3 : Constant  Value=zeros(31,1)  OutDataTypeStr=double  SampleTime=-1
  Input Param. for forwardKinematics and  computeJacobians 4 : Constant  Value=zeros(31,1)  OutDataTypeStr=double  SampleTime=-1
  S-Function : S-Function  FunctionName=robotState  Parameters=val,robotname,localname  EnableBusSupport=off  mask{val=3, robotname=robotName, localname=localName}
      mask prompts: val "Value"; robotname "Robot Name (icub - icubSim)"; localname "Module Name"
  Terminator{1..2,4..5} (4 alike) : Terminator
  dqRad : Terminator
  massMatrix : Terminator
  massMatrix1 : Terminator
  qRad : Terminator
  x : Terminator
  Jacobian : Outport
  wires:
  S-Function/7 -> Terminator5/1
  S-Function/6 -> Terminator4/1
  S-Function/5 -> massMatrix/1
  S-Function/2 -> dqRad/1
  S-Function/1 -> qRad/1
  S-Function/3 -> x/1
  "Input Param. for forwardKinematics and  computeJacobians "/1 -> S-Function/1
  S-Function/4 -> Jacobian/1
  Input Param. for forwardKinematics and  computeJacobians 1/1 -> S-Function/2
  S-Function/8 -> massMatrix1/1
  S-Function/9 -> Terminator1/1
  S-Function/10 -> Terminator2/1
  Input Param. for forwardKinematics and  computeJacobians 2/1 -> S-Function/3
  Input Param. for forwardKinematics and  computeJacobians 3/1 -> S-Function/4
  Input Param. for forwardKinematics and  computeJacobians 4/1 -> S-Function/5

== system WBCLibrary/wholeBodyModel/Jacobians/Left Foot Jacobian/Left Foot  Jacobian1 ==
  "Input Param. for forwardKinematics and  computeJacobians " : Constant  OutDataTypeStr=int8
  Input Param. for forwardKinematics and  computeJacobians 1 : Constant  Value=zeros(25,1)  OutDataTypeStr=double  SampleTime=-1
  Input Param. for forwardKinematics and  computeJacobians 2 : Constant  Value=zeros(25+16,1)  OutDataTypeStr=double  SampleTime=-1
  Input Param. for forwardKinematics and  computeJacobians 3 : Constant  Value=zeros(31,1)  OutDataTypeStr=double  SampleTime=-1
  Input Param. for forwardKinematics and  computeJacobians 4 : Constant  Value=zeros(31,1)  OutDataTypeStr=double  SampleTime=-1
  S-Function : S-Function  FunctionName=robotState  Parameters=val,robotname,localname  EnableBusSupport=off  mask{val=3, robotname=robotName, localname=localName}
      mask prompts: val "Value"; robotname "Robot Name (icub - icubSim)"; localname "Module Name"
  Terminator1 : Terminator
  Terminator2 : Terminator
  Terminator3 : Terminator
  dqrad : Terminator
  dqrad1 : Terminator
  dqrad2 : Terminator
  massMatrix : Terminator
  massMatrix1 : Terminator
  qrad : Terminator
  Jacobian : Outport
  wires:
  Input Param. for forwardKinematics and  computeJacobians 1/1 -> S-Function/2
  S-Function/2 -> dqrad/1
  S-Function/1 -> qrad/1
  S-Function/3 -> Terminator1/1
  "Input Param. for forwardKinematics and  computeJacobians "/1 -> S-Function/1
  S-Function/4 -> Jacobian/1
  S-Function/5 -> massMatrix/1
  S-Function/6 -> Terminator3/1
  S-Function/7 -> dqrad1/1
  S-Function/8 -> massMatrix1/1
  S-Function/9 -> Terminator2/1
  S-Function/10 -> dqrad2/1
  Input Param. for forwardKinematics and  computeJacobians 2/1 -> S-Function/3
  Input Param. for forwardKinematics and  computeJacobians 3/1 -> S-Function/4
  Input Param. for forwardKinematics and  computeJacobians 4/1 -> S-Function/5

== system WBCLibrary/wholeBodyModel/Jacobians/Right Foot Jacobian/Right Foot  Jacobian1 ==
  "Input Param. for forwardKinematics and  computeJacobians " : Constant  Value=0  OutDataTypeStr=int8  SampleTime=-1
  Input Param. for forwardKinematics and  computeJacobians 1 : Constant  Value=zeros(25,1)  OutDataTypeStr=double  SampleTime=-1
  Input Param. for forwardKinematics and  computeJacobians 2 : Constant  Value=zeros(25+16,1)  OutDataTypeStr=double  SampleTime=-1
  Input Param. for forwardKinematics and  computeJacobians 3 : Constant  Value=zeros(31,1)  OutDataTypeStr=double  SampleTime=-1
  Input Param. for forwardKinematics and  computeJacobians 4 : Constant  Value=zeros(31,1)  OutDataTypeStr=double  SampleTime=-1
  S-Function : S-Function  FunctionName=robotState  Parameters=val,robotname,localname  EnableBusSupport=off  mask{val=3, robotname=robotName, localname=localName}
      mask prompts: val "Value"; robotname "Robot Name (icub - icubSim)"; localname "Module Name"
  Terminator{1..5} (5 alike) : Terminator
  dqRad : Terminator
  massMatrix : Terminator
  qRad : Terminator
  x : Terminator
  Jacobian : Outport
  wires:
  Input Param. for forwardKinematics and  computeJacobians 1/1 -> S-Function/2
  S-Function/4 -> Jacobian/1
  "Input Param. for forwardKinematics and  computeJacobians "/1 -> S-Function/1
  S-Function/3 -> x/1
  S-Function/1 -> qRad/1
  S-Function/2 -> dqRad/1
  S-Function/5 -> massMatrix/1
  S-Function/6 -> Terminator4/1
  S-Function/7 -> Terminator5/1
  S-Function/8 -> Terminator1/1
  S-Function/9 -> Terminator2/1
  S-Function/10 -> Terminator3/1
  Input Param. for forwardKinematics and  computeJacobians 2/1 -> S-Function/3
  Input Param. for forwardKinematics and  computeJacobians 3/1 -> S-Function/4
  Input Param. for forwardKinematics and  computeJacobians 4/1 -> S-Function/5

== matlab function Utilities/baseVelocity/MATLAB Function ==
  data: JacobRF input double; JacobLF input double; y output double; qD input double
function y = fcn(JacobRF, JacobLF, qD)
%#codegen
y = -pinv(JacobRF*JacobLF*qD)

== matlab function Utilities/DampPinv/Damped Pseudo Inverse ==
  data: mat input double; DPinv output double; sigma input double
function DPinv  = fcn(mat,sigma)
% Economody size svd of mat
[U,S,V] = svd(mat,'econ');
% Damped version of S with sigma
S(S>sigma)=S(S>sigma)./((S(S>sigma)).^2+sigma^2);
% Damped pseudoinverse
DPinv = V*pinv(S)*U';

== matlab function Utilities/TruncPinv/Truncated PseudoInverse ==
  data: mat input double; TPinv output double; tol input double
function TPinv  = fcn(mat,tol)
%#codegen
[U,S,V] = svd(mat,'econ');
% Setting to zero value
% Setting to 1/S(i,i) singular values greater than tol
 S(S>tol)=1./S(S>tol);
 TPinv = V*pinv(S)*U';
